simulink model "systemResponse"  (R2019b)
settings: Solver=VariableStepAuto  StartTime=0.0  StopTime=10  RelTol=1e-3
libraries: simulink x1
settings Model: Creator=63291  LastModifiedBy=63291

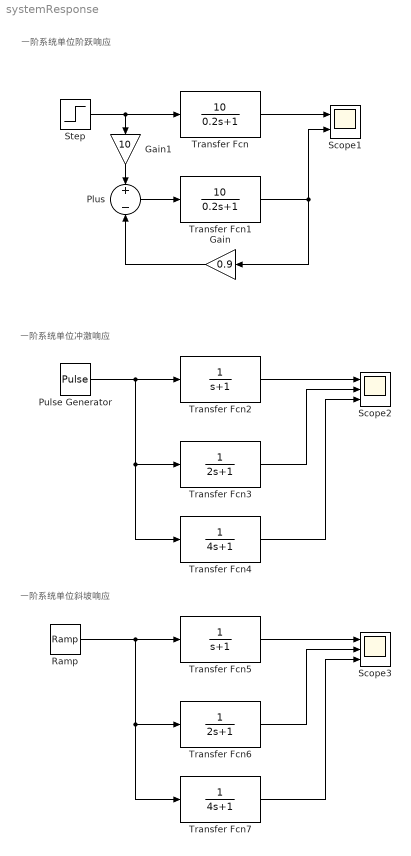
== system systemResponse ==
  note: 一阶系统单位冲激响应
  note: 一阶系统单位阶跃响应
  note: 一阶系统单位斜坡响应
  Gain : Gain  Gain=0.9
  Gain1 : Gain  Gain=10
  Plus : Sum  Inputs=+-
  Pulse Generator : DiscretePulseGenerator  PulseType=Time based  Period=10  PulseWidth=0.0001
  Ramp : simulink/Sources/Ramp  slope=1  start=0  InitialOutput=0
  Scope1 : Scope  NumInputPorts=2
  Scope2 : Scope  NumInputPorts=3
  Scope3 : Scope  NumInputPorts=3
  Step : Step  Time=0  SampleTime=0
  Transfer Fcn : TransferFcn  Numerator=[10]  Denominator=[0.2 1]
  Transfer Fcn1 : TransferFcn  Numerator=[10]  Denominator=[0.2 1]
  Transfer Fcn2 : TransferFcn  Denominator=[1 1]
  Transfer Fcn3 : TransferFcn  Denominator=[2 1]
  Transfer Fcn4 : TransferFcn  Denominator=[4 1]
  Transfer Fcn5 : TransferFcn  Denominator=[1 1]
  Transfer Fcn6 : TransferFcn  Denominator=[2 1]
  Transfer Fcn7 : TransferFcn  Denominator=[4 1]
  wires:
  Step/1 -> Transfer Fcn/1, Gain1/1
  Transfer Fcn/1 -> Scope1/1
  Transfer Fcn1/1 -> Gain/1, Scope1/2
  Gain/1 -> Plus/2
  Gain1/1 -> Plus/1
  Plus/1 -> Transfer Fcn1/1
  Pulse Generator/1 -> Transfer Fcn4/1, Transfer Fcn3/1, Transfer Fcn2/1
  Transfer Fcn2/1 -> Scope2/1
  Transfer Fcn3/1 -> Scope2/2
  Transfer Fcn4/1 -> Scope2/3
  Transfer Fcn7/1 -> Scope3/3
  Transfer Fcn6/1 -> Scope3/2
  Transfer Fcn5/1 -> Scope3/1
  Ramp/1 -> Transfer Fcn5/1, Transfer Fcn6/1, Transfer Fcn7/1
